simulink library "BechamoNasaOpenModels"  (R2024a)
settings: Solver=VariableStepAuto  StartTime=0.0  StopTime=10.0  RelTol=1e-3
values from neighbouring files (symbols this model uses):
  Cl_aileron_wing_1 = Cl_mat.Claileron_wing.axes1.value    [setupMavrik.m]
  Cl_aileron_wing_2 = Cl_mat.Claileron_wing.axes2.value    [setupMavrik.m]
  Cl_aileron_wing_3 = Cl_mat.Claileron_wing.axes3.value    [setupMavrik.m]
  Cl_aileron_wing_val = Cl_mat.Claileron_wing.value    [setupMavrik.m]
  Cl_elevator_tail_1 = Cl_mat.Clelevator_tail.axes1.value    [setupMavrik.m]
  Cl_elevator_tail_2 = Cl_mat.Clelevator_tail.axes2.value    [setupMavrik.m]
  Cl_elevator_tail_3 = Cl_mat.Clelevator_tail.axes3.value    [setupMavrik.m]
  Cl_elevator_tail_val = Cl_mat.Clelevator_tail.value    [setupMavrik.m]
  Cl_flap_wing_1 = Cl_mat.Clflap_wing.axes1.value    [setupMavrik.m]
  Cl_flap_wing_2 = Cl_mat.Clflap_wing.axes2.value    [setupMavrik.m]
  Cl_flap_wing_3 = Cl_mat.Clflap_wing.axes3.value    [setupMavrik.m]
  Cl_flap_wing_val = Cl_mat.Clflap_wing.value    [setupMavrik.m]
  Cl_hover_fuse_1 = Cl_mat.Clhover_fuse.axes1.value    [setupMavrik.m]
  Cl_hover_fuse_2 = Cl_mat.Clhover_fuse.axes2.value    [setupMavrik.m]
  Cl_hover_fuse_3 = Cl_mat.Clhover_fuse.axes3.value    [setupMavrik.m]
  Cl_hover_fuse_val = Cl_mat.Clhover_fuse.value    [setupMavrik.m]
  Cl_rudder_tail_1 = Cl_mat.Clrudder_tail.axes1.value    [setupMavrik.m]
  Cl_rudder_tail_2 = Cl_mat.Clrudder_tail.axes2.value    [setupMavrik.m]
  Cl_rudder_tail_3 = Cl_mat.Clrudder_tail.axes3.value    [setupMavrik.m]
  Cl_rudder_tail_val = Cl_mat.Clrudder_tail.value    [setupMavrik.m]
  Cl_tail_1 = Cl_mat.Cltail.axes1.value    [setupMavrik.m]
  Cl_tail_2 = Cl_mat.Cltail.axes2.value    [setupMavrik.m]
  Cl_tail_3 = Cl_mat.Cltail.axes3.value    [setupMavrik.m]
  Cl_tail_damp_p_1 = Cl_mat.Cltail_damp_p.axes1.value    [setupMavrik.m]
  Cl_tail_damp_p_2 = Cl_mat.Cltail_damp_p.axes2.value    [setupMavrik.m]
  Cl_tail_damp_p_3 = Cl_mat.Cltail_damp_p.axes3.value    [setupMavrik.m]
  Cl_tail_damp_p_val = Cl_mat.Cltail_damp_p.value    [setupMavrik.m]
  Cl_tail_damp_q_1 = Cl_mat.Cltail_damp_q.axes1.value    [setupMavrik.m]
  Cl_tail_damp_q_2 = Cl_mat.Cltail_damp_q.axes2.value    [setupMavrik.m]
  Cl_tail_damp_q_3 = Cl_mat.Cltail_damp_q.axes3.value    [setupMavrik.m]
  Cl_tail_damp_q_val = Cl_mat.Cltail_damp_q.value    [setupMavrik.m]
  Cl_tail_damp_r_1 = Cl_mat.Cltail_damp_r.axes1.value    [setupMavrik.m]
  Cl_tail_damp_r_2 = Cl_mat.Cltail_damp_r.axes2.value    [setupMavrik.m]
  Cl_tail_damp_r_3 = Cl_mat.Cltail_damp_r.axes3.value    [setupMavrik.m]
  Cl_tail_damp_r_val = Cl_mat.Cltail_damp_r.value    [setupMavrik.m]
  Cl_tail_val = Cl_mat.Cltail.value    [setupMavrik.m]
  Cl_wing_1 = Cl_mat.Clwing.axes1.value    [setupMavrik.m]
  Cl_wing_2 = Cl_mat.Clwing.axes2.value    [setupMavrik.m]
  Cl_wing_3 = Cl_mat.Clwing.axes3.value    [setupMavrik.m]
  Cl_wing_damp_p_1 = Cl_mat.Clwing_damp_p.axes1.value    [setupMavrik.m]
  Cl_wing_damp_p_2 = Cl_mat.Clwing_damp_p.axes2.value    [setupMavrik.m]
  Cl_wing_damp_p_3 = Cl_mat.Clwing_damp_p.axes3.value    [setupMavrik.m]
  Cl_wing_damp_p_val = Cl_mat.Clwing_damp_p.value    [setupMavrik.m]
  Cl_wing_damp_q_1 = Cl_mat.Clwing_damp_q.axes1.value    [setupMavrik.m]
  Cl_wing_damp_q_2 = Cl_mat.Clwing_damp_q.axes2.value    [setupMavrik.m]
  Cl_wing_damp_q_3 = Cl_mat.Clwing_damp_q.axes3.value    [setupMavrik.m]
  Cl_wing_damp_q_val = Cl_mat.Clwing_damp_q.value    [setupMavrik.m]
  Cl_wing_damp_r_1 = Cl_mat.Clwing_damp_r.axes1.value    [setupMavrik.m]
  Cl_wing_damp_r_2 = Cl_mat.Clwing_damp_r.axes2.value    [setupMavrik.m]
  Cl_wing_damp_r_3 = Cl_mat.Clwing_damp_r.axes3.value    [setupMavrik.m]
  Cl_wing_damp_r_val = Cl_mat.Clwing_damp_r.value    [setupMavrik.m]
  Cl_wing_val = Cl_mat.Clwing.value    [setupMavrik.m]
  Cm_aileron_wing_1 = Cm_mat.Cmaileron_wing.axes1.value    [setupMavrik.m]
  Cm_aileron_wing_2 = Cm_mat.Cmaileron_wing.axes2.value    [setupMavrik.m]
  Cm_aileron_wing_3 = Cm_mat.Cmaileron_wing.axes3.value    [setupMavrik.m]
  Cm_aileron_wing_val = Cm_mat.Cmaileron_wing.value    [setupMavrik.m]
  Cm_elevator_tail_1 = Cm_mat.Cmelevator_tail.axes1.value    [setupMavrik.m]
  Cm_elevator_tail_2 = Cm_mat.Cmelevator_tail.axes2.value    [setupMavrik.m]
  Cm_elevator_tail_3 = Cm_mat.Cmelevator_tail.axes3.value    [setupMavrik.m]
  Cm_elevator_tail_val = Cm_mat.Cmelevator_tail.value    [setupMavrik.m]
  Cm_flap_wing_1 = Cm_mat.Cmflap_wing.axes1.value    [setupMavrik.m]
  Cm_flap_wing_2 = Cm_mat.Cmflap_wing.axes2.value    [setupMavrik.m]
  Cm_flap_wing_3 = Cm_mat.Cmflap_wing.axes3.value    [setupMavrik.m]
  Cm_flap_wing_val = Cm_mat.Cmflap_wing.value    [setupMavrik.m]
  Cm_hover_fuse_1 = Cm_mat.Cmhover_fuse.axes1.value    [setupMavrik.m]
  Cm_hover_fuse_2 = Cm_mat.Cmhover_fuse.axes2.value    [setupMavrik.m]
  Cm_hover_fuse_3 = Cm_mat.Cmhover_fuse.axes3.value    [setupMavrik.m]
  Cm_hover_fuse_val = Cm_mat.Cmhover_fuse.value    [setupMavrik.m]
  Cm_rudder_tail_1 = Cm_mat.Cmrudder_tail.axes1.value    [setupMavrik.m]
  Cm_rudder_tail_2 = Cm_mat.Cmrudder_tail.axes2.value    [setupMavrik.m]
  Cm_rudder_tail_3 = Cm_mat.Cmrudder_tail.axes3.value    [setupMavrik.m]
  Cm_rudder_tail_val = Cm_mat.Cmrudder_tail.value    [setupMavrik.m]
  Cm_tail_1 = Cm_mat.Cmtail.axes1.value    [setupMavrik.m]
  Cm_tail_2 = Cm_mat.Cmtail.axes2.value    [setupMavrik.m]
  Cm_tail_3 = Cm_mat.Cmtail.axes3.value    [setupMavrik.m]
  Cm_tail_damp_p_1 = Cm_mat.Cmtail_damp_p.axes1.value    [setupMavrik.m]
  Cm_tail_damp_p_2 = Cm_mat.Cmtail_damp_p.axes2.value    [setupMavrik.m]
  Cm_tail_damp_p_3 = Cm_mat.Cmtail_damp_p.axes3.value    [setupMavrik.m]
  Cm_tail_damp_p_val = Cm_mat.Cmtail_damp_p.value    [setupMavrik.m]
  Cm_tail_damp_q_1 = Cm_mat.Cmtail_damp_q.axes1.value    [setupMavrik.m]
  Cm_tail_damp_q_2 = Cm_mat.Cmtail_damp_q.axes2.value    [setupMavrik.m]
  Cm_tail_damp_q_3 = Cm_mat.Cmtail_damp_q.axes3.value    [setupMavrik.m]
  Cm_tail_damp_q_val = Cm_mat.Cmtail_damp_q.value    [setupMavrik.m]
  Cm_tail_damp_r_1 = Cm_mat.Cmtail_damp_r.axes1.value    [setupMavrik.m]
  Cm_tail_damp_r_2 = Cm_mat.Cmtail_damp_r.axes2.value    [setupMavrik.m]
  Cm_tail_damp_r_3 = Cm_mat.Cmtail_damp_r.axes3.value    [setupMavrik.m]
  Cm_tail_damp_r_val = Cm_mat.Cmtail_damp_r.value    [setupMavrik.m]
  Cm_tail_val = Cm_mat.Cmtail.value    [setupMavrik.m]
  Cm_wing_1 = Cm_mat.Cmwing.axes1.value    [setupMavrik.m]
  Cm_wing_2 = Cm_mat.Cmwing.axes2.value    [setupMavrik.m]
  Cm_wing_3 = Cm_mat.Cmwing.axes3.value    [setupMavrik.m]
  Cm_wing_damp_p_1 = Cm_mat.Cmwing_damp_p.axes1.value    [setupMavrik.m]
  Cm_wing_damp_p_2 = Cm_mat.Cmwing_damp_p.axes2.value    [setupMavrik.m]
  Cm_wing_damp_p_3 = Cm_mat.Cmwing_damp_p.axes3.value    [setupMavrik.m]
  Cm_wing_damp_p_val = Cm_mat.Cmwing_damp_p.value    [setupMavrik.m]
  Cm_wing_damp_q_1 = Cm_mat.Cmwing_damp_q.axes1.value    [setupMavrik.m]
  Cm_wing_damp_q_2 = Cm_mat.Cmwing_damp_q.axes2.value    [setupMavrik.m]
  Cm_wing_damp_q_3 = Cm_mat.Cmwing_damp_q.axes3.value    [setupMavrik.m]
  Cm_wing_damp_q_val = Cm_mat.Cmwing_damp_q.value    [setupMavrik.m]
  Cm_wing_damp_r_1 = Cm_mat.Cmwing_damp_r.axes1.value    [setupMavrik.m]
  Cm_wing_damp_r_2 = Cm_mat.Cmwing_damp_r.axes2.value    [setupMavrik.m]
  Cm_wing_damp_r_3 = Cm_mat.Cmwing_damp_r.axes3.value    [setupMavrik.m]
  Cm_wing_damp_r_val = Cm_mat.Cmwing_damp_r.value    [setupMavrik.m]
  Cm_wing_val = Cm_mat.Cmwing.value    [setupMavrik.m]
  Cn_aileron_wing_1 = Cn_mat.Cnaileron_wing.axes1.value    [setupMavrik.m]
  Cn_aileron_wing_2 = Cn_mat.Cnaileron_wing.axes2.value    [setupMavrik.m]
  Cn_aileron_wing_3 = Cn_mat.Cnaileron_wing.axes3.value    [setupMavrik.m]
  Cn_aileron_wing_val = Cn_mat.Cnaileron_wing.value    [setupMavrik.m]
  Cn_elevator_tail_1 = Cn_mat.Cnelevator_tail.axes1.value    [setupMavrik.m]
  Cn_elevator_tail_2 = Cn_mat.Cnelevator_tail.axes2.value    [setupMavrik.m]
  Cn_elevator_tail_3 = Cn_mat.Cnelevator_tail.axes3.value    [setupMavrik.m]
  Cn_elevator_tail_val = Cn_mat.Cnelevator_tail.value    [setupMavrik.m]
  Cn_flap_wing_1 = Cn_mat.Cnflap_wing.axes1.value    [setupMavrik.m]
  Cn_flap_wing_2 = Cn_mat.Cnflap_wing.axes2.value    [setupMavrik.m]
  Cn_flap_wing_3 = Cn_mat.Cnflap_wing.axes3.value    [setupMavrik.m]
  Cn_flap_wing_val = Cn_mat.Cnflap_wing.value    [setupMavrik.m]
  Cn_hover_fuse_1 = Cn_mat.Cnhover_fuse.axes1.value    [setupMavrik.m]
  Cn_hover_fuse_2 = Cn_mat.Cnhover_fuse.axes2.value    [setupMavrik.m]
  Cn_hover_fuse_3 = Cn_mat.Cnhover_fuse.axes3.value    [setupMavrik.m]
  Cn_hover_fuse_val = Cn_mat.Cnhover_fuse.value    [setupMavrik.m]
  ... (+318 more)
libraries: matrix_library x15, shared6dof x1, sharedtransform x1
(part 2 of 19)

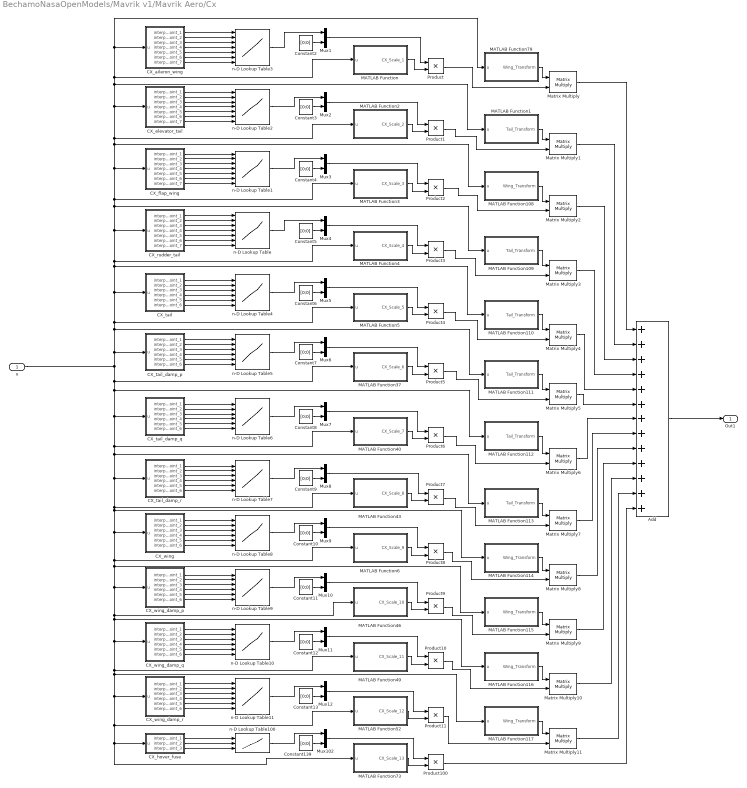
== system BechamoNasaOpenModels/Mavrik v1/Mavrik Aero/Cx ==
  u : Inport
  Add : Sum  Inputs=+++++++++++++
  CX_aileron_wing : MATLAB Function  TreatAsAtomicUnit=on
  CX_elevator_tail : MATLAB Function  TreatAsAtomicUnit=on
  CX_flap_wing : MATLAB Function  TreatAsAtomicUnit=on
  CX_hover_fuse : MATLAB Function  TreatAsAtomicUnit=on
  CX_rudder_tail : MATLAB Function  TreatAsAtomicUnit=on
  CX_tail : MATLAB Function  TreatAsAtomicUnit=on
  CX_tail_damp_p : MATLAB Function  TreatAsAtomicUnit=on
  CX_tail_damp_q : MATLAB Function  TreatAsAtomicUnit=on
  CX_tail_damp_r : MATLAB Function  TreatAsAtomicUnit=on
  CX_wing : MATLAB Function  TreatAsAtomicUnit=on
  CX_wing_damp_p : MATLAB Function  TreatAsAtomicUnit=on
  CX_wing_damp_q : MATLAB Function  TreatAsAtomicUnit=on
  CX_wing_damp_r : MATLAB Function  TreatAsAtomicUnit=on
  Constant{2..13,139} (13 alike) : Constant  Value=[0;0]
  MATLAB Function : MATLAB Function  TreatAsAtomicUnit=on
  MATLAB Function1 : MATLAB Function  TreatAsAtomicUnit=on
  MATLAB Function108 : MATLAB Function  TreatAsAtomicUnit=on
  MATLAB Function109 : MATLAB Function  TreatAsAtomicUnit=on
  MATLAB Function110 : MATLAB Function  TreatAsAtomicUnit=on
  MATLAB Function111 : MATLAB Function  TreatAsAtomicUnit=on
  MATLAB Function112 : MATLAB Function  TreatAsAtomicUnit=on
  MATLAB Function113 : MATLAB Function  TreatAsAtomicUnit=on
  MATLAB Function114 : MATLAB Function  TreatAsAtomicUnit=on
  MATLAB Function115 : MATLAB Function  TreatAsAtomicUnit=on
  MATLAB Function116 : MATLAB Function  TreatAsAtomicUnit=on
  MATLAB Function117 : MATLAB Function  TreatAsAtomicUnit=on
  MATLAB Function2 : MATLAB Function  TreatAsAtomicUnit=on
  MATLAB Function3 : MATLAB Function  TreatAsAtomicUnit=on
  MATLAB Function37 : MATLAB Function  TreatAsAtomicUnit=on
  MATLAB Function4 : MATLAB Function  TreatAsAtomicUnit=on
  MATLAB Function40 : MATLAB Function  TreatAsAtomicUnit=on
  MATLAB Function43 : MATLAB Function  TreatAsAtomicUnit=on
  MATLAB Function46 : MATLAB Function  TreatAsAtomicUnit=on
  MATLAB Function49 : MATLAB Function  TreatAsAtomicUnit=on
  MATLAB Function5 : MATLAB Function  TreatAsAtomicUnit=on
  MATLAB Function52 : MATLAB Function  TreatAsAtomicUnit=on
  MATLAB Function6 : MATLAB Function  TreatAsAtomicUnit=on
  MATLAB Function73 : MATLAB Function  TreatAsAtomicUnit=on
  MATLAB Function79 : MATLAB Function  TreatAsAtomicUnit=on
  Matrix Multiply{,1..11} (12 alike) : Product  Multiplication=Matrix(*)
  Mux{1..12,102} (13 alike) : Mux  Inputs=2
  Product{,1..11,100} (13 alike) : Product
  n-D Lookup Table : Lookup_n-D  NumberOfTableDimensions=7  BreakpointsForDimension1=CX_rudder_tail_1  BreakpointsForDimension2=CX_rudder_tail_2  BreakpointsForDimension3=CX_rudder_tail_3  BreakpointsForDimension4=CX_rudder_tail_4  BreakpointsForDimension5=CX_rudder_tail_5  BreakpointsForDimension6=CX_rudder_tail_6  BreakpointsForDimension7=CX_rudder_tail_7  Table=CX_rudder_tail_val  InternalRulePriority=Speed  OutDataTypeStr=Inherit: Inherit via back propagation  RndMeth=Simplest
      settings: InputPortMap=u0,u1,u2,u3,u4,u5,u6
  n-D Lookup Table1 : Lookup_n-D  NumberOfTableDimensions=7  BreakpointsForDimension1=CX_flap_wing_1  BreakpointsForDimension2=CX_flap_wing_2  BreakpointsForDimension3=CX_flap_wing_3  BreakpointsForDimension4=CX_flap_wing_4  BreakpointsForDimension5=CX_flap_wing_5  BreakpointsForDimension6=CX_flap_wing_6  BreakpointsForDimension7=CX_flap_wing_7  Table=CX_flap_wing_val  InternalRulePriority=Speed  OutDataTypeStr=Inherit: Inherit via back propagation  RndMeth=Simplest
      settings: InputPortMap=u0,u1,u2,u3,u4,u5,u6
  n-D Lookup Table10 : Lookup_n-D  NumberOfTableDimensions=6  BreakpointsForDimension1=CX_wing_damp_q_1  BreakpointsForDimension2=CX_wing_damp_q_2  BreakpointsForDimension3=CX_wing_damp_q_3  BreakpointsForDimension4=CX_wing_damp_q_4  BreakpointsForDimension5=CX_wing_damp_q_5  BreakpointsForDimension6=CX_wing_damp_q_6  BreakpointsForDimension7=CX_flap_wing_7  Table=CX_wing_damp_q_val  InternalRulePriority=Speed  OutDataTypeStr=Inherit: Inherit via back propagation  RndMeth=Simplest
      settings: InputPortMap=u0,u1,u2,u3,u4,u5
  n-D Lookup Table100 : Lookup_n-D  NumberOfTableDimensions=3  BreakpointsForDimension1=CX_hover_fuse_1  BreakpointsForDimension2=CX_hover_fuse_2  BreakpointsForDimension3=CX_hover_fuse_3  BreakpointsForDimension4=CX_wing_damp_r_4  BreakpointsForDimension5=CX_wing_damp_r_5  BreakpointsForDimension6=CX_wing_damp_r_6  BreakpointsForDimension7=CX_flap_wing_7  Table=CX_hover_fuse_val  InternalRulePriority=Speed  OutDataTypeStr=Inherit: Inherit via back propagation  RndMeth=Simplest
      settings: InputPortMap=u0,u1,u2
  n-D Lookup Table11 : Lookup_n-D  NumberOfTableDimensions=6  BreakpointsForDimension1=CX_wing_damp_r_1  BreakpointsForDimension2=CX_wing_damp_r_2  BreakpointsForDimension3=CX_wing_damp_r_3  BreakpointsForDimension4=CX_wing_damp_r_4  BreakpointsForDimension5=CX_wing_damp_r_5  BreakpointsForDimension6=CX_wing_damp_r_6  BreakpointsForDimension7=CX_flap_wing_7  Table=CX_wing_damp_r_val  InternalRulePriority=Speed  OutDataTypeStr=Inherit: Inherit via back propagation  RndMeth=Simplest
      settings: InputPortMap=u0,u1,u2,u3,u4,u5
  n-D Lookup Table2 : Lookup_n-D  NumberOfTableDimensions=7  BreakpointsForDimension1=CX_elevator_tail_1  BreakpointsForDimension2=CX_elevator_tail_2  BreakpointsForDimension3=CX_elevator_tail_3  BreakpointsForDimension4=CX_elevator_tail_4  BreakpointsForDimension5=CX_elevator_tail_5  BreakpointsForDimension6=CX_elevator_tail_6  BreakpointsForDimension7=CX_elevator_tail_7  Table=CX_elevator_tail_val  InternalRulePriority=Speed  OutDataTypeStr=Inherit: Inherit via back propagation  RndMeth=Simplest
      settings: InputPortMap=u0,u1,u2,u3,u4,u5,u6
  n-D Lookup Table3 : Lookup_n-D  NumberOfTableDimensions=7  BreakpointsForDimension1=CX_aileron_wing_1  BreakpointsForDimension2=CX_aileron_wing_2  BreakpointsForDimension3=CX_aileron_wing_3  BreakpointsForDimension4=CX_aileron_wing_4  BreakpointsForDimension5=CX_aileron_wing_5  BreakpointsForDimension6=CX_aileron_wing_6  BreakpointsForDimension7=CX_aileron_wing_7  Table=CX_aileron_wing_val  InternalRulePriority=Speed  OutDataTypeStr=Inherit: Inherit via back propagation  RndMeth=Simplest
      settings: InputPortMap=u0,u1,u2,u3,u4,u5,u6
  n-D Lookup Table4 : Lookup_n-D  NumberOfTableDimensions=6  BreakpointsForDimension1=CX_tail_1  BreakpointsForDimension2=CX_tail_2  BreakpointsForDimension3=CX_tail_3  BreakpointsForDimension4=CX_tail_4  BreakpointsForDimension5=CX_tail_5  BreakpointsForDimension6=CX_tail_6  BreakpointsForDimension7=CX_tail_7  Table=CX_tail_val  InternalRulePriority=Speed  OutDataTypeStr=Inherit: Inherit via back propagation  RndMeth=Simplest
      settings: InputPortMap=u0,u1,u2,u3,u4,u5
  n-D Lookup Table5 : Lookup_n-D  NumberOfTableDimensions=6  BreakpointsForDimension1=CX_tail_damp_p_1  BreakpointsForDimension2=CX_tail_damp_p_2  BreakpointsForDimension3=CX_tail_damp_p_3  BreakpointsForDimension4=CX_tail_damp_p_4  BreakpointsForDimension5=CX_tail_damp_p_5  BreakpointsForDimension6=CX_tail_damp_p_6  BreakpointsForDimension7=CX_tail_7  Table=CX_tail_damp_p_val  InternalRulePriority=Speed  OutDataTypeStr=Inherit: Inherit via back propagation  RndMeth=Simplest
      settings: InputPortMap=u0,u1,u2,u3,u4,u5
  n-D Lookup Table6 : Lookup_n-D  NumberOfTableDimensions=6  BreakpointsForDimension1=CX_tail_damp_q_1  BreakpointsForDimension2=CX_tail_damp_q_2  BreakpointsForDimension3=CX_tail_damp_q_3  BreakpointsForDimension4=CX_tail_damp_q_4  BreakpointsForDimension5=CX_tail_damp_q_5  BreakpointsForDimension6=CX_tail_damp_q_6  BreakpointsForDimension7=CX_tail_7  Table=CX_tail_damp_q_val  InternalRulePriority=Speed  OutDataTypeStr=Inherit: Inherit via back propagation  RndMeth=Simplest
      settings: InputPortMap=u0,u1,u2,u3,u4,u5
  n-D Lookup Table7 : Lookup_n-D  NumberOfTableDimensions=6  BreakpointsForDimension1=CX_tail_damp_r_1  BreakpointsForDimension2=CX_tail_damp_r_2  BreakpointsForDimension3=CX_tail_damp_r_3  BreakpointsForDimension4=CX_tail_damp_r_4  BreakpointsForDimension5=CX_tail_damp_r_5  BreakpointsForDimension6=CX_tail_damp_r_6  BreakpointsForDimension7=CX_tail_7  Table=CX_tail_damp_r_val  InternalRulePriority=Speed  OutDataTypeStr=Inherit: Inherit via back propagation  RndMeth=Simplest
      settings: InputPortMap=u0,u1,u2,u3,u4,u5
  n-D Lookup Table8 : Lookup_n-D  NumberOfTableDimensions=6  BreakpointsForDimension1=CX_wing_1  BreakpointsForDimension2=CX_wing_2  BreakpointsForDimension3=CX_wing_3  BreakpointsForDimension4=CX_wing_4  BreakpointsForDimension5=CX_wing_5  BreakpointsForDimension6=CX_wing_6  BreakpointsForDimension7=CX_flap_wing_7  Table=CX_wing_val  InternalRulePriority=Speed  OutDataTypeStr=Inherit: Inherit via back propagation  RndMeth=Simplest
      settings: InputPortMap=u0,u1,u2,u3,u4,u5
  n-D Lookup Table9 : Lookup_n-D  NumberOfTableDimensions=6  BreakpointsForDimension1=CX_wing_damp_p_1  BreakpointsForDimension2=CX_wing_damp_p_2  BreakpointsForDimension3=CX_wing_damp_p_3  BreakpointsForDimension4=CX_wing_damp_p_4  BreakpointsForDimension5=CX_wing_damp_p_5  BreakpointsForDimension6=CX_wing_damp_p_6  BreakpointsForDimension7=CX_flap_wing_7  Table=CX_wing_damp_p_val  InternalRulePriority=Speed  OutDataTypeStr=Inherit: Inherit via back propagation  RndMeth=Simplest
      settings: InputPortMap=u0,u1,u2,u3,u4,u5
  Out1 : Outport
  wires:
  Constant7/1 -> Mux6/2
  MATLAB Function116/1(Wing_Transform) -> Matrix Multiply10/1
  CX_wing_damp_r/2(interp_point_2) -> n-D Lookup Table11/2
  Constant9/1 -> Mux8/2
  Constant12/1 -> Mux11/2
  CX_tail_damp_r/1(interp_point_1) -> n-D Lookup Table7/1
  CX_wing/5(interp_point_5) -> n-D Lookup Table8/5
  CX_rudder_tail/6(interp_point_6) -> n-D Lookup Table/6
  CX_wing_damp_q/3(interp_point_3) -> n-D Lookup Table10/3
  CX_wing/2(interp_point_2) -> n-D Lookup Table8/2
  CX_aileron_wing/2(interp_point_2) -> n-D Lookup Table3/2
  CX_elevator_tail/7(interp_point_7) -> n-D Lookup Table2/7
  CX_aileron_wing/5(interp_point_5) -> n-D Lookup Table3/5
  Matrix Multiply2/1 -> Add/3
  MATLAB Function/1(CX_Scale_1) -> Product/2
  CX_wing_damp_p/3(interp_point_3) -> n-D Lookup Table9/3
  Product11/1 -> Matrix Multiply11/2
  MATLAB Function4/1(CX_Scale_4) -> Product3/2
  CX_wing_damp_q/4(interp_point_4) -> n-D Lookup Table10/4
  CX_flap_wing/3(interp_point_3) -> n-D Lookup Table1/3
  Matrix Multiply3/1 -> Add/4
  Mux12/1 -> Product11/1
  Matrix Multiply7/1 -> Add/8
  Mux1/1 -> Product/1
  MATLAB Function79/1(Wing_Transform) -> Matrix Multiply/1
  MATLAB Function1/1(Tail_Transform) -> Matrix Multiply1/1
  Matrix Multiply6/1 -> Add/7
  CX_tail_damp_q/2(interp_point_2) -> n-D Lookup Table6/2
  CX_wing_damp_r/3(interp_point_3) -> n-D Lookup Table11/3
  MATLAB Function117/1(Wing_Transform) -> Matrix Multiply11/1
  u/1 -> MATLAB Function73/1(u), CX_hover_fuse/1(u), MATLAB Function52/1(u), CX_wing_damp_r/1(u), MATLAB Function117/1(u), MATLAB Function49/1(u), CX_wing_damp_q/1(u), MATLAB Function116/1(u), MATLAB Function46/1(u), CX_wing_damp_p/1(u), MATLAB Function115/1(u), MATLAB Function6/1(u), CX_wing/1(u), MATLAB Function114/1(u), MATLAB Function43/1(u), CX_tail_damp_r/1(u), MATLAB Function113/1(u), MATLAB Function40/1(u), CX_tail_damp_q/1(u), MATLAB Function112/1(u), MATLAB Function37/1(u), CX_tail_damp_p/1(u), MATLAB Function111/1(u), MATLAB Function5/1(u), MATLAB Function110/1(u), MATLAB Function4/1(u), MATLAB Function109/1(u), MATLAB Function3/1(u), MATLAB Function2/1(u), MATLAB Function1/1(u), MATLAB Function79/1(u), CX_aileron_wing/1(u), MATLAB Function/1(u), CX_elevator_tail/1(u), MATLAB Function108/1(u), CX_flap_wing/1(u), CX_rudder_tail/1(u), CX_tail/1(u)
  CX_wing_damp_q/1(interp_point_1) -> n-D Lookup Table10/1
  CX_rudder_tail/1(interp_point_1) -> n-D Lookup Table/1
  Matrix Multiply4/1 -> Add/5
  CX_wing_damp_p/5(interp_point_5) -> n-D Lookup Table9/5
  CX_wing_damp_q/5(interp_point_5) -> n-D Lookup Table10/5
  CX_wing/1(interp_point_1) -> n-D Lookup Table8/1
  CX_elevator_tail/1(interp_point_1) -> n-D Lookup Table2/1
  CX_tail_damp_q/6(interp_point_6) -> n-D Lookup Table6/6
  MATLAB Function49/1(CX_Scale_11) -> Product10/2
  Constant10/1 -> Mux9/2
  CX_wing_damp_p/1(interp_point_1) -> n-D Lookup Table9/1
  CX_wing_damp_p/2(interp_point_2) -> n-D Lookup Table9/2
  CX_wing_damp_p/6(interp_point_6) -> n-D Lookup Table9/6
  CX_rudder_tail/3(interp_point_3) -> n-D Lookup Table/3
  CX_tail_damp_p/4(interp_point_4) -> n-D Lookup Table5/4
  Mux7/1 -> Product6/1
  CX_hover_fuse/2(interp_point_2) -> n-D Lookup Table100/2
  CX_elevator_tail/5(interp_point_5) -> n-D Lookup Table2/5
  CX_tail/2(interp_point_2) -> n-D Lookup Table4/2
  CX_wing_damp_r/1(interp_point_1) -> n-D Lookup Table11/1
  CX_flap_wing/6(interp_point_6) -> n-D Lookup Table1/6
  Mux3/1 -> Product2/1
  CX_wing_damp_p/4(interp_point_4) -> n-D Lookup Table9/4
  Mux6/1 -> Product5/1
  CX_aileron_wing/7(interp_point_7) -> n-D Lookup Table3/7
  Constant139/1 -> Mux102/2
  Matrix Multiply10/1 -> Add/11
  CX_tail_damp_q/1(interp_point_1) -> n-D Lookup Table6/1
  Matrix Multiply/1 -> Add/1
  MATLAB Function115/1(Wing_Transform) -> Matrix Multiply9/1
  n-D Lookup Table4/1 -> Mux5/1
  CX_aileron_wing/6(interp_point_6) -> n-D Lookup Table3/6
  Constant4/1 -> Mux3/2
  CX_tail_damp_p/2(interp_point_2) -> n-D Lookup Table5/2
  Product100/1 -> Add/13
  CX_tail_damp_p/3(interp_point_3) -> n-D Lookup Table5/3
  MATLAB Function37/1(CX_Scale_6) -> Product5/2
  CX_elevator_tail/6(interp_point_6) -> n-D Lookup Table2/6
  Mux102/1 -> Product100/1
  CX_hover_fuse/1(interp_point_1) -> n-D Lookup Table100/1
  MATLAB Function108/1(Wing_Transform) -> Matrix Multiply2/1
  MATLAB Function111/1(Tail_Transform) -> Matrix Multiply5/1
  Constant6/1 -> Mux5/2
  MATLAB Function112/1(Tail_Transform) -> Matrix Multiply6/1
  Matrix Multiply8/1 -> Add/9
  Product5/1 -> Matrix Multiply5/2
  Mux2/1 -> Product1/1
  CX_tail_damp_r/4(interp_point_4) -> n-D Lookup Table7/4
  MATLAB Function73/1(CX_Scale_13) -> Product100/2
  n-D Lookup Table100/1 -> Mux102/1
  CX_tail/1(interp_point_1) -> n-D Lookup Table4/1
  Matrix Multiply1/1 -> Add/2
  CX_tail_damp_q/3(interp_point_3) -> n-D Lookup Table6/3
  CX_hover_fuse/3(interp_point_3) -> n-D Lookup Table100/3
  n-D Lookup Table2/1 -> Mux2/1
  CX_rudder_tail/2(interp_point_2) -> n-D Lookup Table/2
  CX_wing_damp_q/2(interp_point_2) -> n-D Lookup Table10/2
  CX_flap_wing/7(interp_point_7) -> n-D Lookup Table1/7
  CX_flap_wing/1(interp_point_1) -> n-D Lookup Table1/1
  CX_rudder_tail/4(interp_point_4) -> n-D Lookup Table/4
  CX_flap_wing/2(interp_point_2) -> n-D Lookup Table1/2
  CX_elevator_tail/2(interp_point_2) -> n-D Lookup Table2/2
  MATLAB Function3/1(CX_Scale_3) -> Product2/2
  MATLAB Function2/1(CX_Scale_2) -> Product1/2
  CX_rudder_tail/5(interp_point_5) -> n-D Lookup Table/5
  Product6/1 -> Matrix Multiply6/2
  CX_flap_wing/4(interp_point_4) -> n-D Lookup Table1/4
  n-D Lookup Table11/1 -> Mux12/1
  n-D Lookup Table/1 -> Mux4/1
  CX_aileron_wing/1(interp_point_1) -> n-D Lookup Table3/1
  CX_aileron_wing/3(interp_point_3) -> n-D Lookup Table3/3
  CX_elevator_tail/4(interp_point_4) -> n-D Lookup Table2/4
  CX_tail/6(interp_point_6) -> n-D Lookup Table4/6
  n-D Lookup Table5/1 -> Mux6/1
  CX_tail/5(interp_point_5) -> n-D Lookup Table4/5
  CX_tail_damp_p/6(interp_point_6) -> n-D Lookup Table5/6
  CX_tail_damp_q/4(interp_point_4) -> n-D Lookup Table6/4
  CX_wing/3(interp_point_3) -> n-D Lookup Table8/3
  CX_tail_damp_p/5(interp_point_5) -> n-D Lookup Table5/5
  Constant8/1 -> Mux7/2
  CX_tail_damp_p/1(interp_point_1) -> n-D Lookup Table5/1
  Product4/1 -> Matrix Multiply4/2
  MATLAB Function113/1(Tail_Transform) -> Matrix Multiply7/1
  MATLAB Function114/1(Wing_Transform) -> Matrix Multiply8/1
  Product9/1 -> Matrix Multiply9/2
  Product8/1 -> Matrix Multiply8/2
  Product7/1 -> Matrix Multiply7/2
  Matrix Multiply5/1 -> Add/6
  n-D Lookup Table1/1 -> Mux3/1
  Mux4/1 -> Product3/1
  Constant13/1 -> Mux12/2
  Constant11/1 -> Mux10/2
  Constant3/1 -> Mux2/2
  n-D Lookup Table7/1 -> Mux8/1
  n-D Lookup Table9/1 -> Mux10/1
  n-D Lookup Table6/1 -> Mux7/1
  n-D Lookup Table10/1 -> Mux11/1
  Mux5/1 -> Product4/1
  Mux9/1 -> Product8/1
  Mux10/1 -> Product9/1
  Mux11/1 -> Product10/1
  Product/1 -> Matrix Multiply/2
  Mux8/1 -> Product7/1
  CX_tail_damp_r/6(interp_point_6) -> n-D Lookup Table7/6
  CX_tail_damp_r/5(interp_point_5) -> n-D Lookup Table7/5
  CX_aileron_wing/4(interp_point_4) -> n-D Lookup Table3/4
  Constant2/1 -> Mux1/2
  CX_wing/4(interp_point_4) -> n-D Lookup Table8/4
  CX_tail/3(interp_point_3) -> n-D Lookup Table4/3
  MATLAB Function5/1(CX_Scale_5) -> Product4/2
  n-D Lookup Table3/1 -> Mux1/1
  CX_tail_damp_r/3(interp_point_3) -> n-D Lookup Table7/3
  MATLAB Function40/1(CX_Scale_7) -> Product6/2
  MATLAB Function43/1(CX_Scale_8) -> Product7/2
  CX_wing_damp_r/5(interp_point_5) -> n-D Lookup Table11/5
  MATLAB Function46/1(CX_Scale_10) -> Product9/2
  MATLAB Function52/1(CX_Scale_12) -> Product11/2
  CX_tail_damp_q/5(interp_point_5) -> n-D Lookup Table6/5
  CX_wing_damp_r/4(interp_point_4) -> n-D Lookup Table11/4
  Constant5/1 -> Mux4/2
  Matrix Multiply9/1 -> Add/10
  CX_wing/6(interp_point_6) -> n-D Lookup Table8/6
  CX_flap_wing/5(interp_point_5) -> n-D Lookup Table1/5
  Matrix Multiply11/1 -> Add/12
  CX_elevator_tail/3(interp_point_3) -> n-D Lookup Table2/3
  CX_tail/4(interp_point_4) -> n-D Lookup Table4/4
  CX_tail_damp_r/2(interp_point_2) -> n-D Lookup Table7/2
  CX_rudder_tail/7(interp_point_7) -> n-D Lookup Table/7
  CX_wing_damp_r/6(interp_point_6) -> n-D Lookup Table11/6
  Product2/1 -> Matrix Multiply2/2
  Product1/1 -> Matrix Multiply1/2
  MATLAB Function110/1(Tail_Transform) -> Matrix Multiply4/1
  n-D Lookup Table8/1 -> Mux9/1
  Product3/1 -> Matrix Multiply3/2
  MATLAB Function6/1(CX_Scale_9) -> Product8/2
  Product10/1 -> Matrix Multiply10/2
  CX_wing_damp_q/6(interp_point_6) -> n-D Lookup Table10/6
  MATLAB Function109/1(Tail_Transform) -> Matrix Multiply3/1
  Add/1 -> Out1/1

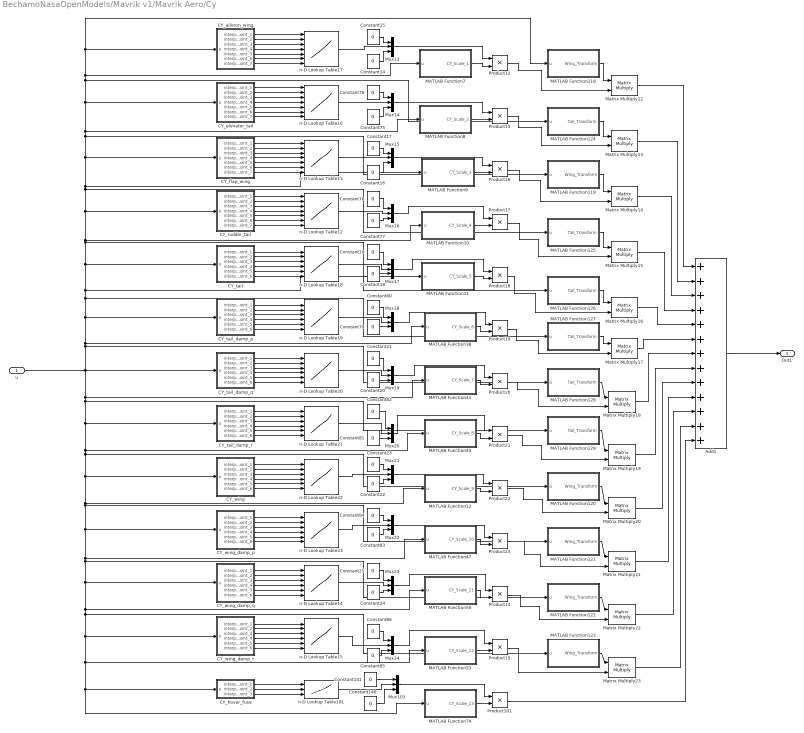
== system BechamoNasaOpenModels/Mavrik v1/Mavrik Aero/Cy ==
  u : Inport
  Add1 : Sum  Inputs=+++++++++++++
  CY_aileron_wing : MATLAB Function  TreatAsAtomicUnit=on
  CY_elevator_tail : MATLAB Function  TreatAsAtomicUnit=on
  CY_flap_wing : MATLAB Function  TreatAsAtomicUnit=on
  CY_hover_fuse : MATLAB Function  TreatAsAtomicUnit=on
  CY_rudder_tail : MATLAB Function  TreatAsAtomicUnit=on
  CY_tail : MATLAB Function  TreatAsAtomicUnit=on
  CY_tail_damp_p : MATLAB Function  TreatAsAtomicUnit=on
  CY_tail_damp_q : MATLAB Function  TreatAsAtomicUnit=on
  CY_tail_damp_r : MATLAB Function  TreatAsAtomicUnit=on
  CY_wing : MATLAB Function  TreatAsAtomicUnit=on
  CY_wing_damp_p : MATLAB Function  TreatAsAtomicUnit=on
  CY_wing_damp_q : MATLAB Function  TreatAsAtomicUnit=on
  CY_wing_damp_r : MATLAB Function  TreatAsAtomicUnit=on
  Constant{14..25,75..86,140..141} (26 alike) : Constant  Value=0
  MATLAB Function10 : MATLAB Function  TreatAsAtomicUnit=on
  MATLAB Function11 : MATLAB Function  TreatAsAtomicUnit=on
  MATLAB Function118 : MATLAB Function  TreatAsAtomicUnit=on
  MATLAB Function119 : MATLAB Function  TreatAsAtomicUnit=on
  MATLAB Function12 : MATLAB Function  TreatAsAtomicUnit=on
  MATLAB Function120 : MATLAB Function  TreatAsAtomicUnit=on
  MATLAB Function121 : MATLAB Function  TreatAsAtomicUnit=on
  MATLAB Function122 : MATLAB Function  TreatAsAtomicUnit=on
  MATLAB Function123 : MATLAB Function  TreatAsAtomicUnit=on
  MATLAB Function124 : MATLAB Function  TreatAsAtomicUnit=on
  MATLAB Function125 : MATLAB Function  TreatAsAtomicUnit=on
  MATLAB Function126 : MATLAB Function  TreatAsAtomicUnit=on
  MATLAB Function127 : MATLAB Function  TreatAsAtomicUnit=on
  MATLAB Function128 : MATLAB Function  TreatAsAtomicUnit=on
  MATLAB Function129 : MATLAB Function  TreatAsAtomicUnit=on
  MATLAB Function38 : MATLAB Function  TreatAsAtomicUnit=on
  MATLAB Function41 : MATLAB Function  TreatAsAtomicUnit=on
  MATLAB Function44 : MATLAB Function  TreatAsAtomicUnit=on
  MATLAB Function47 : MATLAB Function  TreatAsAtomicUnit=on
  MATLAB Function50 : MATLAB Function  TreatAsAtomicUnit=on
  MATLAB Function53 : MATLAB Function  TreatAsAtomicUnit=on
  MATLAB Function7 : MATLAB Function  TreatAsAtomicUnit=on
  MATLAB Function74 : MATLAB Function  TreatAsAtomicUnit=on
  MATLAB Function8 : MATLAB Function  TreatAsAtomicUnit=on
  MATLAB Function9 : MATLAB Function  TreatAsAtomicUnit=on
  Matrix Multiply{12..23} (12 alike) : Product  Multiplication=Matrix(*)
  Mux{13..24,103} (13 alike) : Mux  Inputs=3
  Product{12..23,101} (13 alike) : Product
  n-D Lookup Table101 : Lookup_n-D  NumberOfTableDimensions=3  BreakpointsForDimension1=CY_hover_fuse_1  BreakpointsForDimension2=CY_hover_fuse_2  BreakpointsForDimension3=CY_hover_fuse_3  BreakpointsForDimension4=CX_wing_damp_r_4  BreakpointsForDimension5=CX_wing_damp_r_5  BreakpointsForDimension6=CX_wing_damp_r_6  BreakpointsForDimension7=CX_flap_wing_7  Table=CY_hover_fuse_val  InternalRulePriority=Speed  OutDataTypeStr=Inherit: Inherit via back propagation  RndMeth=Simplest
      settings: InputPortMap=u0,u1,u2
  n-D Lookup Table12 : Lookup_n-D  NumberOfTableDimensions=7  BreakpointsForDimension1=CY_rudder_tail_1  BreakpointsForDimension2=CY_rudder_tail_2  BreakpointsForDimension3=CY_rudder_tail_3  BreakpointsForDimension4=CY_rudder_tail_4  BreakpointsForDimension5=CY_rudder_tail_5  BreakpointsForDimension6=CY_rudder_tail_6  BreakpointsForDimension7=CY_rudder_tail_7  Table=CY_rudder_tail_val  InternalRulePriority=Speed  OutDataTypeStr=Inherit: Inherit via back propagation  RndMeth=Simplest
      settings: InputPortMap=u0,u1,u2,u3,u4,u5,u6
  n-D Lookup Table13 : Lookup_n-D  NumberOfTableDimensions=7  BreakpointsForDimension1=CY_flap_wing_1  BreakpointsForDimension2=CY_flap_wing_2  BreakpointsForDimension3=CY_flap_wing_3  BreakpointsForDimension4=CY_flap_wing_4  BreakpointsForDimension5=CY_flap_wing_5  BreakpointsForDimension6=CY_flap_wing_6  BreakpointsForDimension7=CY_flap_wing_7  Table=CY_flap_wing_val  InternalRulePriority=Speed  OutDataTypeStr=Inherit: Inherit via back propagation  RndMeth=Simplest
      settings: InputPortMap=u0,u1,u2,u3,u4,u5,u6
  n-D Lookup Table14 : Lookup_n-D  NumberOfTableDimensions=6  BreakpointsForDimension1=CY_wing_damp_q_1  BreakpointsForDimension2=CY_wing_damp_q_2  BreakpointsForDimension3=CY_wing_damp_q_3  BreakpointsForDimension4=CY_wing_damp_q_4  BreakpointsForDimension5=CY_wing_damp_q_5  BreakpointsForDimension6=CY_wing_damp_q_6  BreakpointsForDimension7=CX_flap_wing_7  Table=CY_wing_damp_q_val  InternalRulePriority=Speed  OutDataTypeStr=Inherit: Inherit via back propagation  RndMeth=Simplest
      settings: InputPortMap=u0,u1,u2,u3,u4,u5
  n-D Lookup Table15 : Lookup_n-D  NumberOfTableDimensions=6  BreakpointsForDimension1=CY_wing_damp_r_1  BreakpointsForDimension2=CY_wing_damp_r_2  BreakpointsForDimension3=CY_wing_damp_r_3  BreakpointsForDimension4=CY_wing_damp_r_4  BreakpointsForDimension5=CY_wing_damp_r_5  BreakpointsForDimension6=CY_wing_damp_r_6  BreakpointsForDimension7=CX_flap_wing_7  Table=CY_wing_damp_r_val  InternalRulePriority=Speed  OutDataTypeStr=Inherit: Inherit via back propagation  RndMeth=Simplest
      settings: InputPortMap=u0,u1,u2,u3,u4,u5
  n-D Lookup Table16 : Lookup_n-D  NumberOfTableDimensions=7  BreakpointsForDimension1=CY_elevator_tail_1  BreakpointsForDimension2=CY_elevator_tail_2  BreakpointsForDimension3=CY_elevator_tail_3  BreakpointsForDimension4=CY_elevator_tail_4  BreakpointsForDimension5=CY_elevator_tail_5  BreakpointsForDimension6=CY_elevator_tail_6  BreakpointsForDimension7=CY_elevator_tail_7  Table=CY_elevator_tail_val  InternalRulePriority=Speed  OutDataTypeStr=Inherit: Inherit via back propagation  RndMeth=Simplest
      settings: InputPortMap=u0,u1,u2,u3,u4,u5,u6
  n-D Lookup Table17 : Lookup_n-D  NumberOfTableDimensions=7  BreakpointsForDimension1=CY_aileron_wing_1  BreakpointsForDimension2=CY_aileron_wing_2  BreakpointsForDimension3=CY_aileron_wing_3  BreakpointsForDimension4=CX_aileron_wing_4  BreakpointsForDimension5=CY_aileron_wing_5  BreakpointsForDimension6=CY_aileron_wing_6  BreakpointsForDimension7=CY_aileron_wing_7  Table=CY_aileron_wing_val  InternalRulePriority=Speed  OutDataTypeStr=Inherit: Inherit via back propagation  RndMeth=Simplest
      settings: InputPortMap=u0,u1,u2,u3,u4,u5,u6
  n-D Lookup Table18 : Lookup_n-D  NumberOfTableDimensions=6  BreakpointsForDimension1=CX_tail_1  BreakpointsForDimension2=CY_tail_2  BreakpointsForDimension3=CY_tail_3  BreakpointsForDimension4=CY_tail_4  BreakpointsForDimension5=CY_tail_5  BreakpointsForDimension6=CY_tail_6  BreakpointsForDimension7=CX_tail_7  Table=CY_tail_val  InternalRulePriority=Speed  OutDataTypeStr=Inherit: Inherit via back propagation  RndMeth=Simplest
      settings: InputPortMap=u0,u1,u2,u3,u4,u5
  n-D Lookup Table19 : Lookup_n-D  NumberOfTableDimensions=6  BreakpointsForDimension1=CY_tail_damp_p_1  BreakpointsForDimension2=CY_tail_damp_p_2  BreakpointsForDimension3=CY_tail_damp_p_3  BreakpointsForDimension4=CY_tail_damp_p_4  BreakpointsForDimension5=CY_tail_damp_p_5  BreakpointsForDimension6=CY_tail_damp_p_6  BreakpointsForDimension7=CX_tail_7  Table=CY_tail_damp_p_val  InternalRulePriority=Speed  OutDataTypeStr=Inherit: Inherit via back propagation  RndMeth=Simplest
      settings: InputPortMap=u0,u1,u2,u3,u4,u5
  n-D Lookup Table20 : Lookup_n-D  NumberOfTableDimensions=6  BreakpointsForDimension1=CY_tail_damp_q_1  BreakpointsForDimension2=CY_tail_damp_q_2  BreakpointsForDimension3=CY_tail_damp_q_3  BreakpointsForDimension4=CY_tail_damp_q_4  BreakpointsForDimension5=CY_tail_damp_q_5  BreakpointsForDimension6=CY_tail_damp_q_6  BreakpointsForDimension7=CX_tail_7  Table=CY_tail_damp_q_val  InternalRulePriority=Speed  OutDataTypeStr=Inherit: Inherit via back propagation  RndMeth=Simplest
      settings: InputPortMap=u0,u1,u2,u3,u4,u5
  n-D Lookup Table21 : Lookup_n-D  NumberOfTableDimensions=6  BreakpointsForDimension1=CY_tail_damp_r_1  BreakpointsForDimension2=CY_tail_damp_r_2  BreakpointsForDimension3=CY_tail_damp_r_3  BreakpointsForDimension4=CY_tail_damp_r_4  BreakpointsForDimension5=CY_tail_damp_r_5  BreakpointsForDimension6=CY_tail_damp_r_6  BreakpointsForDimension7=CX_tail_7  Table=CY_tail_damp_r_val  InternalRulePriority=Speed  OutDataTypeStr=Inherit: Inherit via back propagation  RndMeth=Simplest
      settings: InputPortMap=u0,u1,u2,u3,u4,u5
  n-D Lookup Table22 : Lookup_n-D  NumberOfTableDimensions=6  BreakpointsForDimension1=CY_wing_1  BreakpointsForDimension2=CY_wing_2  BreakpointsForDimension3=CY_wing_3  BreakpointsForDimension4=CY_wing_4  BreakpointsForDimension5=CY_wing_5  BreakpointsForDimension6=CY_wing_6  BreakpointsForDimension7=CX_flap_wing_7  Table=CY_wing_val  InternalRulePriority=Speed  OutDataTypeStr=Inherit: Inherit via back propagation  RndMeth=Simplest
      settings: InputPortMap=u0,u1,u2,u3,u4,u5
  n-D Lookup Table23 : Lookup_n-D  NumberOfTableDimensions=6  BreakpointsForDimension1=CY_wing_damp_p_1  BreakpointsForDimension2=CY_wing_damp_p_2  BreakpointsForDimension3=CY_wing_damp_p_3  BreakpointsForDimension4=CY_wing_damp_p_4  BreakpointsForDimension5=CY_wing_damp_p_5  BreakpointsForDimension6=CY_wing_damp_p_6  BreakpointsForDimension7=CX_flap_wing_7  Table=CY_wing_damp_p_val  InternalRulePriority=Speed  OutDataTypeStr=Inherit: Inherit via back propagation  RndMeth=Simplest
      settings: InputPortMap=u0,u1,u2,u3,u4,u5
  Out1 : Outport
  wires:
  Product14/1 -> Matrix Multiply22/2
  CY_tail/1(interp_point_1) -> n-D Lookup Table18/1
  CY_elevator_tail/1(interp_point_1) -> n-D Lookup Table16/1
  Mux19/1 -> Product20/1
  Product22/1 -> Matrix Multiply20/2
  CY_tail_damp_p/6(interp_point_6) -> n-D Lookup Table19/6
  Product16/1 -> Matrix Multiply14/2
  Matrix Multiply19/1 -> Add1/8
  CY_tail_damp_p/2(interp_point_2) -> n-D Lookup Table19/2
  Mux15/1 -> Product16/1
  CY_wing_damp_p/3(interp_point_3) -> n-D Lookup Table23/3
  MATLAB Function129/1(Tail_Transform) -> Matrix Multiply19/1
  CY_tail_damp_q/6(interp_point_6) -> n-D Lookup Table20/6
  CY_wing_damp_p/1(interp_point_1) -> n-D Lookup Table23/1
  Mux13/1 -> Product12/1
  MATLAB Function122/1(Wing_Transform) -> Matrix Multiply22/1
  CY_aileron_wing/2(interp_point_2) -> n-D Lookup Table17/2
  CY_wing_damp_r/4(interp_point_4) -> n-D Lookup Table15/4
  Mux22/1 -> Product23/1
  CY_wing_damp_r/6(interp_point_6) -> n-D Lookup Table15/6
  CY_wing/5(interp_point_5) -> n-D Lookup Table22/5
  Matrix Multiply12/1 -> Add1/1
  CY_tail_damp_r/5(interp_point_5) -> n-D Lookup Table21/5
  CY_tail_damp_q/1(interp_point_1) -> n-D Lookup Table20/1
  CY_wing/3(interp_point_3) -> n-D Lookup Table22/3
  n-D Lookup Table101/1 -> Mux103/2
  MATLAB Function126/1(Tail_Transform) -> Matrix Multiply16/1
  CY_wing/4(interp_point_4) -> n-D Lookup Table22/4
  CY_aileron_wing/7(interp_point_7) -> n-D Lookup Table17/7
  CY_tail_damp_q/3(interp_point_3) -> n-D Lookup Table20/3
  Mux103/1 -> Product101/1
  Matrix Multiply21/1 -> Add1/10
  Mux24/1 -> Product15/1
  Product19/1 -> Matrix Multiply17/2
  CY_rudder_tail/5(interp_point_5) -> n-D Lookup Table12/5
  CY_wing_damp_p/6(interp_point_6) -> n-D Lookup Table23/6
  CY_wing_damp_q/6(interp_point_6) -> n-D Lookup Table14/6
  Matrix Multiply23/1 -> Add1/12
  Matrix Multiply20/1 -> Add1/9
  CY_wing_damp_r/1(interp_point_1) -> n-D Lookup Table15/1
  CY_tail/3(interp_point_3) -> n-D Lookup Table18/3
  Mux18/1 -> Product19/1
  CY_flap_wing/5(interp_point_5) -> n-D Lookup Table13/5
  CY_hover_fuse/2(interp_point_2) -> n-D Lookup Table101/2
  CY_wing_damp_p/2(interp_point_2) -> n-D Lookup Table23/2
  CY_wing_damp_q/5(interp_point_5) -> n-D Lookup Table14/5
  MATLAB Function120/1(Wing_Transform) -> Matrix Multiply20/1
  MATLAB Function12/1(CY_Scale_9) -> Product22/2
  CY_tail_damp_p/3(interp_point_3) -> n-D Lookup Table19/3
  CY_wing_damp_q/3(interp_point_3) -> n-D Lookup Table14/3
  Matrix Multiply13/1 -> Add1/2
  MATLAB Function128/1(Tail_Transform) -> Matrix Multiply18/1
  Mux17/1 -> Product18/1
  CY_tail_damp_r/4(interp_point_4) -> n-D Lookup Table21/4
  CY_tail_damp_p/4(interp_point_4) -> n-D Lookup Table19/4
  CY_flap_wing/4(interp_point_4) -> n-D Lookup Table13/4
  CY_tail_damp_p/1(interp_point_1) -> n-D Lookup Table19/1
  MATLAB Function123/1(Wing_Transform) -> Matrix Multiply23/1
  CY_elevator_tail/2(interp_point_2) -> n-D Lookup Table16/2
  CY_rudder_tail/6(interp_point_6) -> n-D Lookup Table12/6
  CY_wing/6(interp_point_6) -> n-D Lookup Table22/6
  MATLAB Function74/1(CY_Scale_13) -> Product101/2
  CY_tail/6(interp_point_6) -> n-D Lookup Table18/6
  CY_tail/5(interp_point_5) -> n-D Lookup Table18/5
  CY_flap_wing/6(interp_point_6) -> n-D Lookup Table13/6
  CY_wing_damp_q/1(interp_point_1) -> n-D Lookup Table14/1
  Add1/1 -> Out1/1
  CY_aileron_wing/4(interp_point_4) -> n-D Lookup Table17/4
  n-D Lookup Table22/1 -> Mux21/2
  CY_elevator_tail/4(interp_point_4) -> n-D Lookup Table16/4
  MATLAB Function7/1(CY_Scale_1) -> Product12/2
  CY_tail_damp_q/4(interp_point_4) -> n-D Lookup Table20/4
  MATLAB Function8/1(CY_Scale_2) -> Product13/2
  Constant20/1 -> Mux19/3
  MATLAB Function53/1(CY_Scale_12) -> Product15/2
  n-D Lookup Table18/1 -> Mux17/2
  MATLAB Function9/1(CY_Scale_3) -> Product16/2
  CY_rudder_tail/7(interp_point_7) -> n-D Lookup Table12/7
  CY_tail_damp_q/2(interp_point_2) -> n-D Lookup Table20/2
  Product20/1 -> Matrix Multiply18/2
  MATLAB Function125/1(Tail_Transform) -> Matrix Multiply15/1
  MATLAB Function124/1(Tail_Transform) -> Matrix Multiply13/1
  CY_tail_damp_q/5(interp_point_5) -> n-D Lookup Table20/5
  CY_aileron_wing/6(interp_point_6) -> n-D Lookup Table17/6
  MATLAB Function11/1(CY_Scale_5) -> Product18/2
  MATLAB Function47/1(CY_Scale_10) -> Product23/2
  CY_aileron_wing/5(interp_point_5) -> n-D Lookup Table17/5
  Constant141/1 -> Mux103/1
  CY_hover_fuse/1(interp_point_1) -> n-D Lookup Table101/1
  Product101/1 -> Add1/13
  CY_tail_damp_r/1(interp_point_1) -> n-D Lookup Table21/1
  CY_elevator_tail/6(interp_point_6) -> n-D Lookup Table16/6
  n-D Lookup Table13/1 -> Mux15/2
  n-D Lookup Table12/1 -> Mux16/2
  Matrix Multiply16/1 -> Add1/5
  Constant75/1 -> Mux14/3
  Constant15/1 -> Mux13/1
  Constant76/1 -> Mux14/1
  n-D Lookup Table16/1 -> Mux14/2
  CY_tail_damp_r/3(interp_point_3) -> n-D Lookup Table21/3
  CY_tail/2(interp_point_2) -> n-D Lookup Table18/2
  CY_tail_damp_r/6(interp_point_6) -> n-D Lookup Table21/6
  Constant80/1 -> Mux18/1
  Constant19/1 -> Mux17/1
  Constant79/1 -> Mux18/3
  Constant18/1 -> Mux17/3
  n-D Lookup Table21/1 -> Mux20/2
  Product12/1 -> Matrix Multiply12/2
  Constant78/1 -> Mux16/1
  Constant82/1 -> Mux20/1
  n-D Lookup Table20/1 -> Mux19/2
  Constant81/1 -> Mux20/3
  Product17/1 -> Matrix Multiply15/2
  Constant21/1 -> Mux19/1
  Constant22/1 -> Mux21/3
  Constant86/1 -> Mux24/1
  CY_wing_damp_r/5(interp_point_5) -> n-D Lookup Table15/5
  Constant85/1 -> Mux24/3
  Constant24/1 -> Mux23/3
  Constant25/1 -> Mux23/1
  Constant83/1 -> Mux22/3
  Constant84/1 -> Mux22/1
  MATLAB Function119/1(Wing_Transform) -> Matrix Multiply14/1
  Constant23/1 -> Mux21/1
  n-D Lookup Table15/1 -> Mux24/2
  CY_aileron_wing/1(interp_point_1) -> n-D Lookup Table17/1
  Matrix Multiply17/1 -> Add1/6
  Product15/1 -> Matrix Multiply23/2
  Product13/1 -> Matrix Multiply13/2
  n-D Lookup Table17/1 -> Mux13/2
  Constant14/1 -> Mux13/3
  Mux21/1 -> Product22/1
  CY_wing_damp_p/5(interp_point_5) -> n-D Lookup Table23/5
  Mux23/1 -> Product14/1
  MATLAB Function121/1(Wing_Transform) -> Matrix Multiply21/1
  CY_wing_damp_p/4(interp_point_4) -> n-D Lookup Table23/4
  MATLAB Function127/1(Tail_Transform) -> Matrix Multiply17/1
  CY_wing_damp_r/3(interp_point_3) -> n-D Lookup Table15/3
  CY_flap_wing/3(interp_point_3) -> n-D Lookup Table13/3
  Product23/1 -> Matrix Multiply21/2
  MATLAB Function50/1(CY_Scale_11) -> Product14/2
  CY_hover_fuse/3(interp_point_3) -> n-D Lookup Table101/3
  CY_wing_damp_q/4(interp_point_4) -> n-D Lookup Table14/4
  Matrix Multiply22/1 -> Add1/11
  Constant16/1 -> Mux15/3
  MATLAB Function10/1(CY_Scale_4) -> Product17/2
  Product18/1 -> Matrix Multiply16/2
  CY_tail_damp_r/2(interp_point_2) -> n-D Lookup Table21/2
  CY_rudder_tail/2(interp_point_2) -> n-D Lookup Table12/2
  CY_elevator_tail/3(interp_point_3) -> n-D Lookup Table16/3
  Constant77/1 -> Mux16/3
  n-D Lookup Table23/1 -> Mux22/2
  Mux20/1 -> Product21/1
  CY_rudder_tail/4(interp_point_4) -> n-D Lookup Table12/4
  MATLAB Function44/1(CY_Scale_8) -> Product21/2
  MATLAB Function38/1(CY_Scale_6) -> Product19/2
  MATLAB Function41/1(CY_Scale_7) -> Product20/2
  CY_wing/1(interp_point_1) -> n-D Lookup Table22/1
  CY_wing_damp_r/2(interp_point_2) -> n-D Lookup Table15/2
  CY_rudder_tail/1(interp_point_1) -> n-D Lookup Table12/1
  CY_aileron_wing/3(interp_point_3) -> n-D Lookup Table17/3
  Mux14/1 -> Product13/1
  Matrix Multiply14/1 -> Add1/3
  CY_tail/4(interp_point_4) -> n-D Lookup Table18/4
  CY_elevator_tail/5(interp_point_5) -> n-D Lookup Table16/5
  CY_tail_damp_p/5(interp_point_5) -> n-D Lookup Table19/5
  CY_flap_wing/2(interp_point_2) -> n-D Lookup Table13/2
  CY_wing/2(interp_point_2) -> n-D Lookup Table22/2
  CY_flap_wing/1(interp_point_1) -> n-D Lookup Table13/1
  CY_elevator_tail/7(interp_point_7) -> n-D Lookup Table16/7
  CY_wing_damp_q/2(interp_point_2) -> n-D Lookup Table14/2
  Matrix Multiply15/1 -> Add1/4
  Constant140/1 -> Mux103/3
  Matrix Multiply18/1 -> Add1/7
  MATLAB Function118/1(Wing_Transform) -> Matrix Multiply12/1
  Mux16/1 -> Product17/1
  n-D Lookup Table14/1 -> Mux23/2
  Product21/1 -> Matrix Multiply19/2
  Constant17/1 -> Mux15/1
  n-D Lookup Table19/1 -> Mux18/2
  CY_rudder_tail/3(interp_point_3) -> n-D Lookup Table12/3
  CY_flap_wing/7(interp_point_7) -> n-D Lookup Table13/7
  u/1 -> MATLAB Function41/1(u), MATLAB Function129/1(u), CY_tail_damp_r/1(u), MATLAB Function44/1(u), MATLAB Function120/1(u), CY_wing/1(u), MATLAB Function12/1(u), MATLAB Function121/1(u), CY_wing_damp_p/1(u), MATLAB Function47/1(u), MATLAB Function122/1(u), CY_wing_damp_q/1(u), MATLAB Function50/1(u), MATLAB Function123/1(u), CY_wing_damp_r/1(u), MATLAB Function53/1(u), CY_hover_fuse/1(u), MATLAB Function74/1(u), MATLAB Function128/1(u), MATLAB Function38/1(u), CY_tail_damp_p/1(u), MATLAB Function127/1(u), MATLAB Function11/1(u), CY_tail/1(u), MATLAB Function126/1(u), MATLAB Function10/1(u), MATLAB Function125/1(u), MATLAB Function9/1(u), CY_flap_wing/1(u), MATLAB Function119/1(u), MATLAB Function8/1(u), CY_elevator_tail/1(u), MATLAB Function124/1(u), MATLAB Function7/1(u), CY_aileron_wing/1(u), MATLAB Function118/1(u), CY_rudder_tail/1(u), CY_tail_damp_q/1(u)
